simulink model "Torque_Control_ETR07"  (R2017b)
settings: Solver=FixedStepAuto  StartTime=0.0  StopTime=10.0  RelTol=1e-3
libraries: simulink x15, dspstat3 x1
(part 2 of 5)

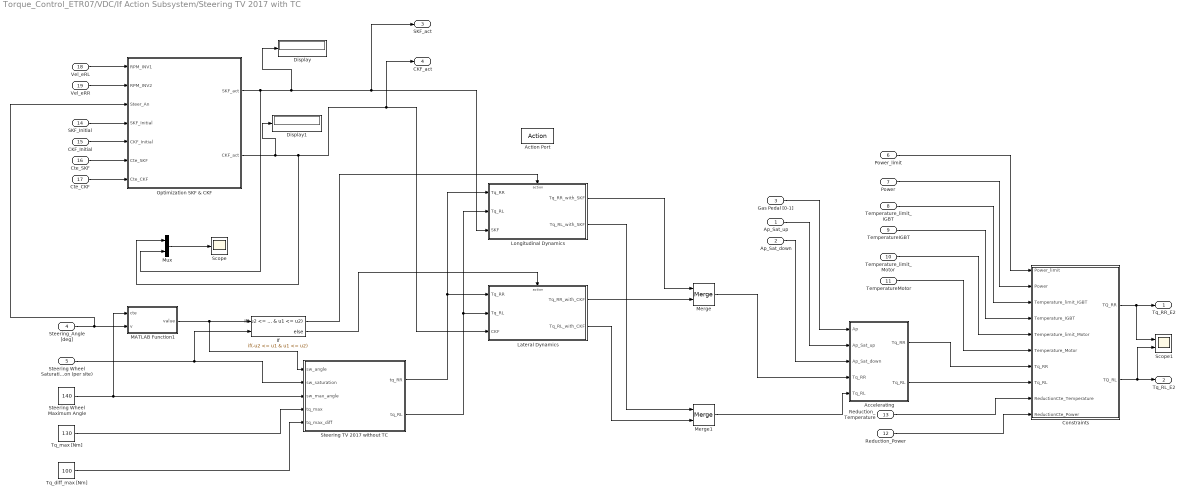
== system Torque_Control_ETR07/VDC/If Action Subsystem/Steering TV 2017 with TC ==
  "Ap_Sat_up " : Inport
  Ap_Sat_down : Inport  Port=2
  Gas Pedal [0-1] : Inport  Port=3
  Steering_Angle [deg] : Inport  Port=4
  "Steering Wheel Saturation (per site) " : Inport  Port=5
  Power_limit : Inport  Port=6
  Power : Inport  Port=7
  Temperature_limit_IGBT : Inport  Port=8
  TemperatureIGBT : Inport  Port=9
  Temperature_limit_Motor : Inport  Port=10
  TemperatureMotor : Inport  Port=11
  Reduction_Power : Inport  Port=12
  Reduction_Temperature : Inport  Port=13
  SKF_Initial : Inport  Port=14
  CKF_Initial : Inport  Port=15
  Cte_SKF : Inport  Port=16
  Cte_CKF : Inport  Port=17
  Vel_eRL : Inport  Port=18
  Vel_eRR : Inport  Port=19
  Action Port : ActionPort  ActionType=elseif
  Accelerating : Subsystem
  Constraints : Subsystem
  Display : Display
  Display1 : Display
  If : If  NumInputs=2  IfExpression=-u2 <= u1 & u1 <= u2
  Lateral Dynamics : Subsystem  TreatAsAtomicUnit=on
  Longitudinal Dynamics : Subsystem  TreatAsAtomicUnit=on
  MATLAB Function1 : MATLAB Function  TreatAsAtomicUnit=on
  Merge : Merge
  Merge1 : Merge
  Mux : Mux  Inputs=2
  Optimization SKF & CKF : Subsystem
  Scope : Scope
  Scope1 : Scope  NumInputPorts=2
  Steering TV 2017 without TC : MATLAB Function  TreatAsAtomicUnit=on
  Steering Wheel Maximum Angle : Constant  Value=140
  Tq_diff_max [Nm] : Constant  Value=100
  Tq_max [Nm] : Constant  Value=130
  Tq_RR_E2 : Outport
  Tq_RL_E2 : Outport  Port=2
  SKF_act : Outport  Port=3
  CKF_act : Outport  Port=4
  wires:
  Gas Pedal [0-1]/1 -> Accelerating/1(Ap)
  "Ap_Sat_up "/1 -> Accelerating/2("Ap_Sat_up ")
  Ap_Sat_down/1 -> Accelerating/3(Ap_Sat_down)
  Tq_max [Nm]/1 -> Steering TV 2017 without TC/4(tq_max)
  Tq_diff_max [Nm]/1 -> Steering TV 2017 without TC/5(tq_max_diff)
  Steering Wheel Maximum Angle/1 -> Steering TV 2017 without TC/3(sw_max_angle), MATLAB Function1/1(cte)
  "Steering Wheel Saturation (per site) "/1 -> If/2, Steering TV 2017 without TC/2(sw_saturation)
  Steering TV 2017 without TC/1(tq_RR) -> Lateral Dynamics/1(Tq_RR), Longitudinal Dynamics/1(Tq_RR)
  Steering TV 2017 without TC/2(tq_RL) -> Lateral Dynamics/2(Tq_RL), Longitudinal Dynamics/2(Tq_RL)
  Power_limit/1 -> Constraints/1(Power_limit)
  Power/1 -> Constraints/2(Power)
  Temperature_limit_IGBT/1 -> Constraints/3(Temperature_limit_IGBT)
  TemperatureIGBT/1 -> Constraints/4(Temperature_IGBT)
  Reduction_Temperature/1 -> Constraints/9(ReductionCte_Temperature)
  Reduction_Power/1 -> Constraints/10(ReductionCte_Power)
  Constraints/1(TQ_RR) -> Scope1/1, Tq_RR_E2/1
  Constraints/2(TQ_RL) -> Scope1/2, Tq_RL_E2/1
  Accelerating/2(Tq_RL) -> Constraints/8(Tq_RL)
  Accelerating/1("Tq_RR ") -> Constraints/7(Tq_RR)
  MATLAB Function1/1(value) -> Steering TV 2017 without TC/1(sw_angle), If/1
  Temperature_limit_Motor/1 -> Constraints/5(Temperature_limit_Motor)
  TemperatureMotor/1 -> Constraints/6(Temperature_Motor)
  Optimization SKF & CKF/2(CKF_act) -> Display1/1, Mux/1, Lateral Dynamics/3(CKF), CKF_act/1
  SKF_Initial/1 -> Optimization SKF & CKF/4(SKF_Initial)
  Mux/1 -> Scope/1
  Cte_SKF/1 -> Optimization SKF & CKF/6(Cte_SKF)
  Vel_eRL/1 -> Optimization SKF & CKF/1(RPM_INV1)
  Vel_eRR/1 -> Optimization SKF & CKF/2(RPM_INV2)
  Optimization SKF & CKF/1(SKF_act) -> SKF_act/1, Longitudinal Dynamics/3(SKF), Display/1, Mux/2
  Steering_Angle [deg]/1 -> MATLAB Function1/2(v), Optimization SKF & CKF/3(Steer_An)
  CKF_Initial/1 -> Optimization SKF & CKF/5(CKF_Initial)
  Cte_CKF/1 -> Optimization SKF & CKF/7(Cte_CKF)
  If/1 -> Longitudinal Dynamics/Action
  Lateral Dynamics/2(Tq_RL_with_CKF) -> Merge1/2
  If/2 -> Lateral Dynamics/Action
  Longitudinal Dynamics/2(Tq_RL_with_SKF) -> Merge1/1
  Longitudinal Dynamics/1(Tq_RR_with_SKF) -> Merge/1
  Lateral Dynamics/1(Tq_RR_with_CKF) -> Merge/2
  Merge/1 -> Accelerating/4(Tq_RR)
  Merge1/1 -> Accelerating/5("Tq_RL ")

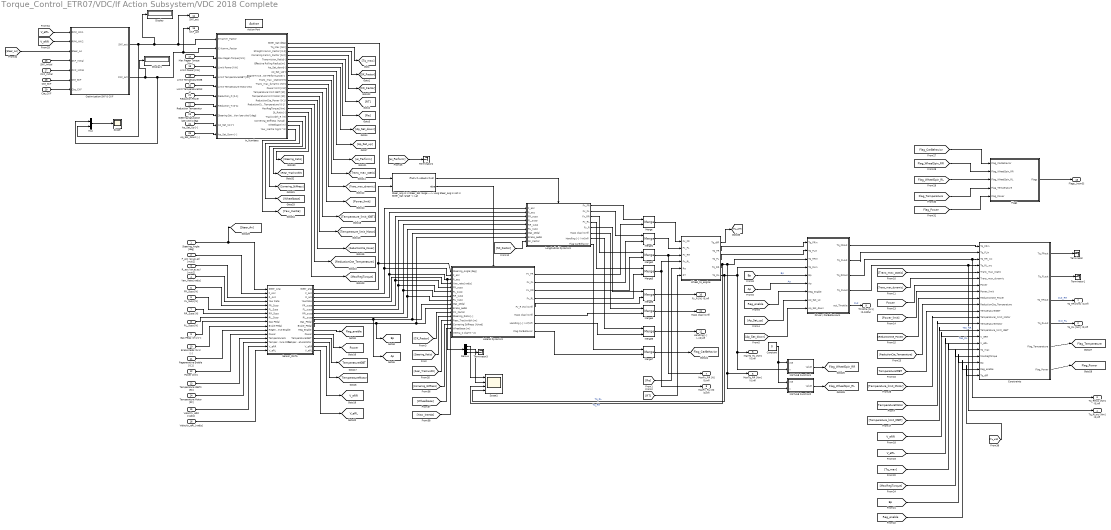
== system Torque_Control_ETR07/VDC/If Action Subsystem/VDC 2018 Complete ==
  Steering_Angle [deg] : Inport
  F_acc (ax,ay,az) [m/s2] : Inport  Port=2
  R_acc (ax,ay,az) [m/s2] : Inport  Port=3
  Yaw_Rate [rad/s] : Inport  Port=4
  FR_Susp [N] : Inport  Port=5
  FL_Susp [N] : Inport  Port=6
  RR_Susp [N] : Inport  Port=7
  RL_Susp [N] : Inport  Port=8
  Gas Pedal (0-1) [-] : Inport  Port=9
  Brake Pedal (0-1) [-] : Inport  Port=10
  Regenerative Enable [0,1] : Inport  Port=11
  Power [kW] : Inport  Port=12
  Temperature IGBTs [ºC] : Inport  Port=13
  Temperature Motor [ºC] : Inport  Port=14
  Velocity_eRR [rad/s] : Inport  Port=15
  Velocity_eRL [rad/s] : Inport  Port=16
  Max Regen Torque [Nm] : Inport  Port=17
  Limit Power [kW] : Inport  Port=18
  Limit TemperatureIGBT : Inport  Port=19
  Limit TemperatureMotor : Inport  Port=20
  Reduction Power : Inport  Port=21
  Reduction Temperature : Inport  Port=22
  Steering Saturation (per site) [deg] : Inport  Port=23
  Ap_Sat_Up [-] : Inport  Port=24
  Ap_Sat_Down [-] : Inport  Port=25
  SKF_Initial : Inport  Port=26
  CKF_Initial : Inport  Port=27
  Cte_SKF : Inport  Port=28
  Cte_CKF : Inport  Port=29
  Action Port : ActionPort  ActionType=then
  Constant : Constant  Value=0
  Constraints : Subsystem
  Demux : Demux  Outputs=3
  Display : Display
  Display1 : Display
  Driver / CarBehaviours : Subsystem
  Flags : Subsystem
  In_Numbers : Subsystem
  Lateral Dynamics : Subsystem  TreatAsAtomicUnit=on
  Longitudinal Dynamics : Subsystem  TreatAsAtomicUnit=on
  MATLAB Function1 : MATLAB Function  TreatAsAtomicUnit=on
  MATLAB Function2 : MATLAB Function  TreatAsAtomicUnit=on
  Merge{,1..7} (8 alike) : Merge
  Mux : Mux  Inputs=2
  Optimization SKF & CKF : Subsystem
  Scope : Scope
  Scope1 : Scope  NumInputPorts=4
  Sensor_DATA : Subsystem
  "Steer_ang is in Steer_Sat range ---> Long Steer_ang is not in Steer_Sat range -> Lat " : If  NumInputs=2  IfExpression=u2>=-u1&u2<=u1
  Terminator{,1..3} (4 alike) : Terminator
  Wheel_to_engine : Subsystem
  Tq_RR [Nm] (0,inf) : Outport
  Tq_RL [Nm] (0,inf) : Outport  Port=2
  Tq_RRwc [Nm] (0,inf) : Outport  Port=3
  Tq_RLwc [Nm] (0,inf) : Outport  Port=4
  MaxTq_RR [Nm] (0,inf) : Outport  Port=5
  MaxTq_RL [Nm] (0,inf) : Outport  Port=6
  MaxFx_RR [N] (0,inf) : Outport  Port=7
  MaxFx_RL [N] (0,inf) : Outport  Port=8
  Throttle [0-1] (0-100%) : Outport  Port=9
  Fy_R [N] (0,inf) : Outport  Port=10
  Mass [kg] (0,inf) : Outport  Port=11
  Handling [-] (-inf,inf) : Outport  Port=12
  Flags_[num5] : Outport  Port=13
  SKF_act : Outport  Port=14
  CKF_act : Outport  Port=15
  tag scope: Ap=global, Bp=global, Flag_CarBehavior=global, Flag_Power=global, Flag_Temperature=global, Flag_WheelSpin_RL=global, Flag_WheelSpin_RR=global, Power=global, Reg_enable=global, TemperatureIGBT=global, TemperatureMotor=global, V_eRL=global, V_eRR=global
  wires:
  "Steer_ang is in Steer_Sat range ---> Long Steer_ang is not in Steer_Sat range -> Lat "/1 -> Longitudinal Dynamics/Action
  "Steer_ang is in Steer_Sat range ---> Long Steer_ang is not in Steer_Sat range -> Lat "/2 -> Lateral Dynamics/Action
  Sensor_DATA/8(RL_susp) -> Longitudinal Dynamics/6(RL_susp), Lateral Dynamics/8(RL_susp)
  In_Numbers/3(Straight Kamm_Factor [0-2]) -> [SK_Factor]
  In_Numbers/1(Steer_Sat [deg]) -> "Steer_ang is in Steer_Sat range ---> Long Steer_ang is not in Steer_Sat range -> Lat "/1
  In_Numbers/2(Tq_Max [Nm]) -> [Tq_max]
  Sensor_DATA/9(Gas_Pedal) -> [Ap], Lateral Dynamics/9(Gas_pedal), Longitudinal Dynamics/7(Gas_pedal)
  In_Numbers/6(Effective Rolling Radius[m]) -> [Re]
  In_Numbers/5(Transmision_Ratio[-]) -> [RT]
  Sensor_DATA/7(RR_susp) -> Longitudinal Dynamics/5(RR_susp), Lateral Dynamics/7(RR_susp)
  In_Numbers/8(Ap_Sat_up[-]) -> [Ap_Sat_up]
  In_Numbers/7(Ap_Sat_down[-]) -> [Ap_Sat_down]
  Driver / CarBehaviours/3(Tq_RRout) -> Tq_RRwc [Nm] (0,inf)/1, Constraints/3(Tq_RR_wc)  "Teo_RR"
  Sensor_DATA/2(F_acc) -> Longitudinal Dynamics/1(F_acc), Lateral Dynamics/2(F_acc)
  Sensor_DATA/3(R_acc) -> Longitudinal Dynamics/2(R_acc), Demux/1, Lateral Dynamics/3(R_acc)
  Sensor_DATA/10(Brake_Pedal) -> [Bp], Lateral Dynamics/10(Brake_pedal), Longitudinal Dynamics/8(Brake_pedal)
  Sensor_DATA/6(FL_susp) -> Longitudinal Dynamics/4(FL_susp), Lateral Dynamics/6(FL_susp)
  Sensor_DATA/11(Reg_Enable) -> [Reg_enable]
  Sensor_DATA/5(FR_susp) -> Longitudinal Dynamics/3(FR_susp), Lateral Dynamics/5(FR_susp)
  Sensor_DATA/1(Steer_ang) -> Lateral Dynamics/1(Steering_Angle [deg]), "Steer_ang is in Steer_Sat range ---> Long Steer_ang is not in Steer_Sat range -> Lat "/2
  Wheel_to_engine/5(Tq_RL) -> Scope1/4, MaxTq_RL [Nm] (0,inf)/1, MATLAB Function1/2(v), Driver / CarBehaviours/4("Tq_RLin ")  "Tq_RL"
  [Trans_max_dynamic] -> Constraints/6(Trans_max_dynamic)
  [Power_limit] -> Constraints/8(Power_limit)
  In_Numbers/15(ReductionCte_Power (0-1)) -> [ReductionCte_Power]
  Driver / CarBehaviours/5(out_Throttle) -> Throttle [0-1] (0-100%)/1  "Out"
  Wheel_to_engine/4(Tq_RR) -> Scope1/3, MATLAB Function2/2(v), MaxTq_RR [Nm] (0,inf)/1, Driver / CarBehaviours/3(Tq_RRin)  "Tq_RR"
  Wheel_to_engine/3(Tq_FL) -> Driver / CarBehaviours/2(Tq_FLin)
  In_Numbers/11(Trans_max_dynamic [Nm]) -> [Trans_max_dynamic]
  [Reg_enable] -> Driver / CarBehaviours/7(Reg_enable)
  [ReductionCte_Power] -> Constraints/9(ReductionCte_Power)
  [Ap_Sat_up] -> Driver / CarBehaviours/8(Ap_Sat_up)
  In_Numbers/10(Trans_max _static[Nm]) -> [Trans_max_static]
  [Ap] -> Driver / CarBehaviours/6(Ap)  "Ap"
  [Power] -> Constraints/7(Power)
  In_Numbers/12("Power limit [KW] ") -> [Power_limit]
  [Ap_Sat_down] -> Driver / CarBehaviours/9(Ap_Sat_down)
  Driver / CarBehaviours/4(Tq_RLout) -> Tq_RLwc [Nm] (0,inf)/1, Constraints/4("Tq_RL_wc ")  "Teo_RL"
  Driver / CarBehaviours/2("Tq_FLout ") -> Constraints/2(Tq_FLin)
  Steering_Angle [deg]/1 -> [Steer_An], Sensor_DATA/1(Steer_Ang)
  Wheel_to_engine/2(Tq_FR) -> Driver / CarBehaviours/1(Tq_FRin)
  Driver / CarBehaviours/1(Tq_FRout) -> Constraints/1(Tq_FRin)
  [Trans_max_static] -> Constraints/5("Trans_max_static ")
  [Temperature_limit_IGBT] -> Constraints/14(Temperature_limit_IGBT)
  [Bp] -> Constraints/19(Bp)
  Sensor_DATA/16(V_eRL) -> [V_eRL]
  In_Numbers/17(MaxRegTorque [Nm]) -> [MaxRegTorque]
  [TemperatureIGBT] -> Constraints/11(TemperatureIGBT)
  [Reg_enable] -> Constraints/20(Reg_enable)
  In_Numbers/9(Engine+Inverter Performance[-]) -> [ei_Perform]
  [Bp] -> Driver / CarBehaviours/5(Bp)  "Bp"
  [Tq_max] -> Constraints/17(Tq_max)
  RR_Susp [N]/1 -> Sensor_DATA/7(RR_Susp)
  Power [kW]/1 -> Sensor_DATA/12("Power ")
  Sensor_DATA/12(Power) -> [Power]
  Sensor_DATA/15("V_eRR ") -> [V_eRR]
  [V_eRR] -> Constraints/15(V_eRR)
  Regenerative Enable [0,1]/1 -> Sensor_DATA/11(Regenerative Enable)
  Brake Pedal (0-1) [-]/1 -> Sensor_DATA/10(Brake Pedal)
  [V_eRL] -> Constraints/16(V_eRL)
  In_Numbers/13(Temperature limit IGBT [ºC]) -> [Temperature_limit_IGBT]
  FL_Susp [N]/1 -> Sensor_DATA/6(FL_Susp)
  FR_Susp [N]/1 -> Sensor_DATA/5(FR_Susp)
  R_acc (ax,ay,az) [m/s2]/1 -> Sensor_DATA/3(R_Acc)
  F_acc (ax,ay,az) [m/s2]/1 -> Sensor_DATA/2("F_Acc ")
  RL_Susp [N]/1 -> Sensor_DATA/8(RL_Susp)
  Gas Pedal (0-1) [-]/1 -> Sensor_DATA/9(Gas Pedal)
  Temperature IGBTs [ºC]/1 -> Sensor_DATA/13(TemperatureIN)
  Velocity_eRR [rad/s]/1 -> Sensor_DATA/15(V_eRR)
  Velocity_eRL [rad/s]/1 -> Sensor_DATA/16("V_eRL ")
  Constraints/1(Tq_FRout) -> Terminator/1
  Constraints/2("Tq_FLout ") -> Terminator1/1
  In_Numbers/4(Cornering Kamm_Factor [0-2]) -> [CK_Factor]
  [Re] -> Wheel_to_engine/5(Re)
  [RT] -> Wheel_to_engine/6(RT)
  Merge3/1 -> MaxFx_RL [N] (0,inf)/1, Wheel_to_engine/4("Fx_RL ")
  Merge2/1 -> Wheel_to_engine/3("Fx_RR "), MaxFx_RR [N] (0,inf)/1
  Merge1/1 -> Wheel_to_engine/2("Fx_FL ")
  Max Regen Torque [Nm]/1 -> In_Numbers/3(Max Regen Torque [Nm])
  Limit Power [kW]/1 -> In_Numbers/4(Limit Power [kW])
  Limit TemperatureIGBT/1 -> In_Numbers/5(Limit TemperatureIGBT [ºC])
  Reduction Power/1 -> In_Numbers/7(Reduction_P [0-1])
  [CK_Factor] -> Lateral Dynamics/11(CK_Factor)
  [SK_Factor] -> Longitudinal Dynamics/9(SK_Factor)
  Longitudinal Dynamics/1(Fx_FR) -> Merge/1
  Longitudinal Dynamics/2(Fx_FL) -> Merge1/1
  Longitudinal Dynamics/3("Fx_RR ") -> Merge2/1
  Longitudinal Dynamics/4("Fx_RL ") -> Merge3/1
  Lateral Dynamics/1(Fx_FR) -> Merge/2
  Lateral Dynamics/2(Fx_FL) -> Merge1/2
  Lateral Dynamics/3("Fx_RR ") -> Merge2/2
  Lateral Dynamics/4("Fx_RL ") -> Merge3/2
  Merge/1 -> Wheel_to_engine/1("Fx_FR ")
  Steering Saturation (per site) [deg]/1 -> In_Numbers/9(Steering Saturation (per site) [deg])
  Ap_Sat_Up [-]/1 -> In_Numbers/10(Ap_Sat_Up [-])
  Ap_Sat_Down [-]/1 -> In_Numbers/11(Ap_Sat_Down [-])
  [MaxRegTorque] -> Constraints/18(MaxRegTorque)
  [ei_Perform] -> Terminator2/1
  Merge4/1 -> Mass [kg] (0,inf)/1
  Longitudinal Dynamics/6(Mass [kg] (0,inf)) -> Merge4/1
  Lateral Dynamics/6(" Mass [kg] (0,inf)") -> Merge4/2
  Longitudinal Dynamics/7(Handling [-] (-inf,inf)) -> Merge5/1
  Lateral Dynamics/7(Handling [-] (-inf,inf)) -> Merge5/2
  Merge5/1 -> Handling [-] (-inf,inf)/1
  Merge6/1 -> Fy_R [N] (0,inf)/1
  Lateral Dynamics/5(Fy_R [N] (0,inf)) -> Merge6/2
  Longitudinal Dynamics/5(Fy_R) -> Merge6/1
  In_Numbers/16(ReductionCte_Temperature (0-1)) -> [ReductionCte_Temperature]
  Reduction Temperature/1 -> In_Numbers/8(Reduction_T [0-1])
  [ReductionCte_Temperature] -> Constraints/10(ReductionCte_Temperature)
  Constraints/3(Tq_RRout) -> Tq_RR [Nm] (0,inf)/1  "Out_RR"
  Constraints/4(Tq_RLout) -> Tq_RL [Nm] (0,inf)/1  "Out_RL"
  Temperature Motor [ºC]/1 -> Sensor_DATA/14(Temperature Motor)
  Sensor_DATA/13(TemperatureIGBT) -> [TemperatureIGBT]
  Sensor_DATA/14(TemperatureMotor) -> [TemperatureMotor]
  [TemperatureMotor] -> Constraints/13(TemperatureIMotor)
  [Temperature_limit_Motor] -> Constraints/12(TemperatureI_limit_Motor)
  In_Numbers/14(Temperature limit Motor [ºC]) -> [Temperature_limit_Motor]
  Limit TemperatureMotor/1 -> In_Numbers/6(Limit Temperature Motor [ºC])
  Merge7/1 -> [Flag_CarBehavior]
  Longitudinal Dynamics/8(Flag CarBehavior) -> Merge7/1
  Lateral Dynamics/8(Flag CarBehavior) -> Merge7/2
  MATLAB Function2/1(value) -> [Flag_WheelSpin_RL]
  MATLAB Function1/1(value) -> [Flag_WheelSpin_RR]
  Constant/1 -> MATLAB Function2/1(cte), MATLAB Function1/1(cte)
  Constraints/5(Flag_Temperature) -> [Flag_Temperature]
  Constraints/6(Flag_Power) -> [Flag_Power]
  Flags/1(Flags) -> Flags_[num5]/1
  [Flag_WheelSpin_RL] -> Flags/3(Flag_WheelSpin_RL)
  [Flag_WheelSpin_RR] -> Flags/2(Flag_WheelSpin_RR)
  [Flag_CarBehavior] -> Flags/1(Flag_CarBehavior)
  [Flag_Temperature] -> Flags/4(Flag_Temperature)
  [Flag_Power] -> Flags/5(Flag_Power)
  Optimization SKF & CKF/1(SKF_act) -> In_Numbers/1(S-Kamm_Factor), SKF_act/1, Display/1, Mux/2
  CKF_Initial/1 -> Optimization SKF & CKF/5(CKF_Initial)
  [Steer_An] -> Optimization SKF & CKF/3(Steer_An)
  [V_eRR] -> Optimization SKF & CKF/2(RPM_INV2)
  Cte_SKF/1 -> Optimization SKF & CKF/6(Cte_SKF)
  Cte_CKF/1 -> Optimization SKF & CKF/7(Cte_CKF)
  SKF_Initial/1 -> Optimization SKF & CKF/4(SKF_Initial)
  [V_eRL] -> Optimization SKF & CKF/1(RPM_INV1)
  Optimization SKF & CKF/2(CKF_act) -> Display1/1, Mux/1, In_Numbers/2(C-Kamm_Factor), CKF_act/1
  Mux/1 -> Scope/1
  Yaw_Rate [rad/s]/1 -> Sensor_DATA/4(Yaw Rate)
  Sensor_DATA/4(YawRate) -> Lateral Dynamics/4(Yaw_rate [rad/s])
  In_Numbers/18(St_Ratio [-]) -> [Steering_Ratio]
  [Steering_Ratio] -> Lateral Dynamics/12(Steering_Ratio [-])
  Demux/2 -> Scope1/2
  Demux/1 -> Scope1/1
  Demux/3 -> Terminator3/1
  In_Numbers/19(Trackwidth_R (m)) -> [Rear_Trackwidth]
  In_Numbers/20(Cornering_Stiffness (N/rad)) -> [Cornering_Stiffness]
  In_Numbers/21(Wheelbase (m)) -> [Wheelbase]
  [Rear_Trackwidth] -> Lateral Dynamics/13(Rear_Trackwidth [m])
  [Cornering_Stiffness] -> Lateral Dynamics/14(Cornering Stiffness [N/rad])
  [Wheelbase] -> Lateral Dynamics/15(Wheelbase [m])
  In_Numbers/22(Yaw_Inertia (kg/m^3)) -> [Yaw_Inertia]
  [Yaw_Inertia] -> Lateral Dynamics/16(Inertia_Z [kg*m^2])
  Wheel_to_engine/1(Tq_diff) -> [Tq_diff]
  [Tq_diff] -> Constraints/21(Tq_diff)

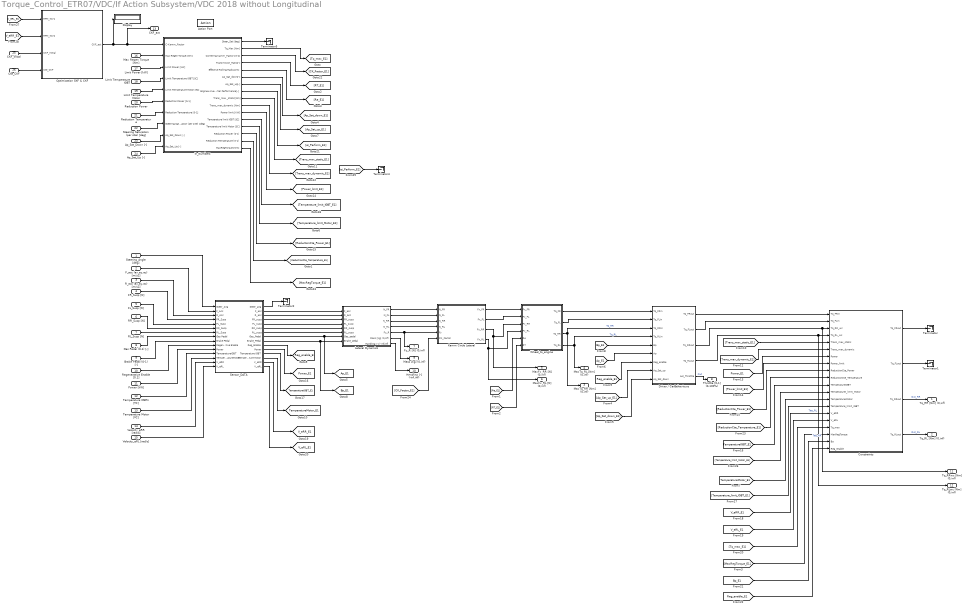
== system Torque_Control_ETR07/VDC/If Action Subsystem/VDC 2018 without Longitudinal ==
  Steering_Angle [deg] : Inport
  F_acc (ax,ay,az) [m/s2] : Inport  Port=2
  R_acc (ax,ay,az) [m/s2] : Inport  Port=3
  FR_Susp [N] : Inport  Port=4
  FL_Susp [N] : Inport  Port=5
  RR_Susp [N] : Inport  Port=6
  RL_Susp [N] : Inport  Port=7
  Gas Pedal (0-1) [-] : Inport  Port=8
  Brake Pedal (0-1) [-] : Inport  Port=9
  Regenerative Enable [0,1] : Inport  Port=10
  Power [kW] : Inport  Port=11
  Temperature IGBTs [ºC] : Inport  Port=12
  Temperature Motor [ºC] : Inport  Port=13
  Velocity_eRR [rad/s] : Inport  Port=14
  Velocity_eRL [rad/s] : Inport  Port=15
  Max Regen Torque [Nm] : Inport  Port=16
  Limit Power [kW] : Inport  Port=17
  Limit Temperature IGBT : Inport  Port=18
  Limit Temperature Motor : Inport  Port=19
  Reduction Power : Inport  Port=20
  Reduction Temperature : Inport  Port=21
  Steering Saturation (per site) [deg] : Inport  Port=22
  Ap_Sat_Down [-] : Inport  Port=23
  Ap_Sat_Up [-] : Inport  Port=24
  CKF_Initial : Inport  Port=25
  Cte_CKF : Inport  Port=26
  Action Port : ActionPort  ActionType=elseif
  Constraints : Subsystem
  Display : Display
  Driver / CarBehaviours : Subsystem
  In_Numbers : Subsystem
  Kamm Circle Lateral : Subsystem
  Lateral Dynamics : Subsystem
  Optimization SKF & CKF : Subsystem
  Sensor_DATA : Subsystem
  Terminator{,1..2,4..5} (5 alike) : Terminator
  Wheel_to_engine : Subsystem
  Tq_RR [Nm] (0,inf) : Outport
  Tq_RL [Nm] (0,inf) : Outport  Port=2
  MaxTq_RR [Nm] (0,inf) : Outport  Port=3
  MaxTq_RL [Nm] (0,inf) : Outport  Port=4
  MaxFx_RR [N] (0,inf) : Outport  Port=5
  MaxFx_RL [N] (0,inf) : Outport  Port=6
  Fy_R [N] (0,inf) : Outport  Port=7
  Throttle [0-1] (0-100%) : Outport  Port=8
  Mass [kg] (0,inf) : Outport  Port=9
  Handling [-] (-inf,inf) : Outport  Port=10
  Tq_RRwc [Nm] (0,inf) : Outport  Port=11
  Tq_RLwc [Nm] (0,inf) : Outport  Port=12
  CKF_act : Outport  Port=13
  tag scope: Ap_E1=global, Bp_E1=global, Power_E1=global, Reg_enable_E1=global, TemperatureIGBT_E1=global, TemperatureMotor_E1=global, V_eRL_E1=global, V_eRR_E1=global
  wires:
  Sensor_DATA/7(RL_susp) -> Lateral Dynamics/6(RL_susp)
  In_Numbers/2(Tq_Max [Nm]) -> [Tq_max_E1]
  Sensor_DATA/8(Gas_Pedal) -> [Ap_E1], Lateral Dynamics/7(Gas_pedal)
  In_Numbers/5(Effective Rolling Radius[m]) -> [Re_E1]
  In_Numbers/4(Transmision_Ratio[-]) -> [RT_E1]
  Sensor_DATA/6(RR_susp) -> Lateral Dynamics/5(RR_susp)
  In_Numbers/7(Ap_Sat_up[-]) -> [Ap_Sat_up_E1]
  In_Numbers/6(Ap_Sat_down[-]) -> [Ap_Sat_down_E1]
  Sensor_DATA/2(F_acc) -> Lateral Dynamics/1(F_acc)
  Sensor_DATA/3(R_acc) -> Lateral Dynamics/2(R_acc)
  Sensor_DATA/9(Brake_Pedal) -> [Bp_E1], Lateral Dynamics/8(Brake_pedal)
  Sensor_DATA/5(FL_susp) -> Lateral Dynamics/4(FL_susp)
  Sensor_DATA/10(Reg_Enable) -> [Reg_enable_E1]
  Sensor_DATA/4(FR_susp) -> Lateral Dynamics/3(FR_susp)
  Wheel_to_engine/4(Tq_RL) -> MaxTq_RL [Nm] (0,inf)/1, Driver / CarBehaviours/4("Tq_RLin ")  "Tq_RL"
  In_Numbers/14(Reduction Power (0-1)) -> [ReductionCte_Power_E1]
  Wheel_to_engine/3(Tq_RR) -> MaxTq_RR [Nm] (0,inf)/1, Driver / CarBehaviours/3(Tq_RRin)  "Tq_RR"
  Wheel_to_engine/2(Tq_FL) -> Driver / CarBehaviours/2(Tq_FLin)
  In_Numbers/10(Trans_max_dynamic [Nm]) -> [Trans_max_dynamic_E1]
  [Reg_enable_E1] -> Driver / CarBehaviours/7(Reg_enable)
  [Ap_Sat_up_E1] -> Driver / CarBehaviours/8(Ap_Sat_up)
  In_Numbers/9(Trans_max _static[Nm]) -> [Trans_max_static_E1]
  [Ap_E1] -> Driver / CarBehaviours/6(Ap)
  In_Numbers/11("Power limit [KW] ") -> [Power_limit_E1]
  [Ap_Sat_down_E1] -> Driver / CarBehaviours/9(Ap_Sat_down)
  Steering_Angle [deg]/1 -> Sensor_DATA/1(Steer_Ang)
  Wheel_to_engine/1(Tq_FR) -> Driver / CarBehaviours/1(Tq_FRin)
  Sensor_DATA/15(V_eRL) -> [V_eRL_E1]
  In_Numbers/16(MaxRegTorque [Nm]) -> [MaxRegTorque_E1]
  In_Numbers/8(Engine+Inverter Performance[-]) -> [ei_Perform_E1]
  [Bp_E1] -> Driver / CarBehaviours/5(Bp)
  Sensor_DATA/12(Temperature IGBT) -> [TemperatureIGBT_E1]
  RR_Susp [N]/1 -> Sensor_DATA/6(RR_Susp)
  Power [kW]/1 -> Sensor_DATA/11("Power ")
  Sensor_DATA/11(Power) -> [Power_E1]
  Sensor_DATA/14("V_eRR ") -> [V_eRR_E1]
  Regenerative Enable [0,1]/1 -> Sensor_DATA/10(Regenerative Enable)
  Brake Pedal (0-1) [-]/1 -> Sensor_DATA/9(Brake Pedal)
  In_Numbers/12(Temperature limit IGBT [ºC]) -> [Temperature_limit_IGBT_E1]
  FL_Susp [N]/1 -> Sensor_DATA/5(FL_Susp)
  FR_Susp [N]/1 -> Sensor_DATA/4(FR_Susp)
  R_acc (ax,ay,az) [m/s2]/1 -> Sensor_DATA/3(R_Acc)
  F_acc (ax,ay,az) [m/s2]/1 -> Sensor_DATA/2("F_Acc ")
  RL_Susp [N]/1 -> Sensor_DATA/7(RL_Susp)
  Gas Pedal (0-1) [-]/1 -> Sensor_DATA/8(Gas Pedal)
  Temperature IGBTs [ºC]/1 -> Sensor_DATA/12(TemperatureIGBT)
  Velocity_eRR [rad/s]/1 -> Sensor_DATA/14(V_eRR)
  Velocity_eRL [rad/s]/1 -> Sensor_DATA/15("V_eRL ")
  Max Regen Torque [Nm]/1 -> In_Numbers/2(Max Regen Torque [Nm])
  Limit Power [kW]/1 -> In_Numbers/3(Limit Power [kW])
  Limit Temperature IGBT/1 -> In_Numbers/4(Limit Temperature IGBT [ºC])
  Reduction Power/1 -> In_Numbers/6(Reduction Power [0-1])
  In_Numbers/3(Cornering Kamm_Factor [0-2]) -> [CK_Factor_E1]
  [Re_E1] -> Wheel_to_engine/5(Re)
  [RT_E1] -> Wheel_to_engine/6(RT)
  Ap_Sat_Up [-]/1 -> In_Numbers/10(Ap_Sat_Up [-])
  Ap_Sat_Down [-]/1 -> In_Numbers/9(Ap_Sat_Down [-])
  Steering Saturation (per site) [deg]/1 -> In_Numbers/8(Steering Saturation (per site) [deg])
  [CK_Factor_E1] -> Kamm Circle Lateral/6(CK_Factor)
  Kamm Circle Lateral/1(Fx_FR) -> Wheel_to_engine/1("Fx_FR ")
  Kamm Circle Lateral/2(Fx_FL) -> Wheel_to_engine/2("Fx_FL ")
  Kamm Circle Lateral/3("Fx_RR ") -> MaxFx_RR [N] (0,inf)/1, Wheel_to_engine/3("Fx_RR ")
  Kamm Circle Lateral/4("Fx_RL ") -> MaxFx_RL [N] (0,inf)/1, Wheel_to_engine/4("Fx_RL ")
  Sensor_DATA/1(Steer_ang) -> Terminator2/1
  Lateral Dynamics/1(N_FR) -> Kamm Circle Lateral/1("N_FR ")
  Lateral Dynamics/2("N_FL ") -> Kamm Circle Lateral/2(N_FL)
  Lateral Dynamics/3("N_RR ") -> Kamm Circle Lateral/3(N_RR)
  Lateral Dynamics/4(N_RL) -> Kamm Circle Lateral/4(N_RL)
  Lateral Dynamics/5(Fy_R) -> Fy_R [N] (0,inf)/1, Kamm Circle Lateral/5(Fy)
  Driver / CarBehaviours/5(out_Throttle) -> Throttle [0-1] (0-100%)/1  "Out"
  [ei_Perform_E1] -> Terminator4/1
  In_Numbers/1(Steer_Sat [deg]) -> Terminator5/1
  Lateral Dynamics/6(Mass [kg] (0,inf)) -> Mass [kg] (0,inf)/1
  Lateral Dynamics/7(Handling [-] (-inf,inf)) -> Handling [-] (-inf,inf)/1
  In_Numbers/15(Reduction Temperature (0-1)) -> [ReductionCte_Temperature_E1]
  Reduction Temperature/1 -> In_Numbers/7(Reduction Temperature [0-1])
  Driver / CarBehaviours/3(Tq_RRout) -> Tq_RRwc [Nm] (0,inf)/1, Constraints/3(Tq_RR_wc)  "Teo_RR"
  [Trans_max_dynamic_E1] -> Constraints/6(Trans_max_dynamic)
  [Power_limit_E1] -> Constraints/8(Power_limit)
  [ReductionCte_Power_E1] -> Constraints/9(ReductionCte_Power)
  [Power_E1] -> Constraints/7(Power)
  Driver / CarBehaviours/4(Tq_RLout) -> Tq_RLwc [Nm] (0,inf)/1, Constraints/4("Tq_RL_wc ")  "Teo_RL"
  Driver / CarBehaviours/2("Tq_FLout ") -> Constraints/2(Tq_FLin)
  Driver / CarBehaviours/1(Tq_FRout) -> Constraints/1(Tq_FRin)
  [Trans_max_static_E1] -> Constraints/5("Trans_max_static ")
  [Temperature_limit_IGBT_E1] -> Constraints/14(Temperature_limit_IGBT)
  [Bp_E1] -> Constraints/19(Bp)
  [TemperatureIGBT_E1] -> Constraints/11(TemperatureIGBT)
  [Reg_enable_E1] -> Constraints/20(Reg_enable)
  [Tq_max_E1] -> Constraints/17(Tq_max)
  [V_eRR_E1] -> Constraints/15(V_eRR)
  [V_eRL_E1] -> Constraints/16(V_eRL)
  Constraints/1(Tq_FRout) -> Terminator/1
  Constraints/2("Tq_FLout ") -> Terminator1/1
  [MaxRegTorque_E1] -> Constraints/18(MaxRegTorque)
  [ReductionCte_Temperature_E1] -> Constraints/10(ReductionCte_Temperature)
  Constraints/3(Tq_RRout) -> Tq_RR [Nm] (0,inf)/1  "Out_RR"
  Constraints/4(Tq_RLout) -> Tq_RL [Nm] (0,inf)/1  "Out_RL"
  [TemperatureMotor_E1] -> Constraints/13(TemperatureIMotor)
  [Temperature_limit_Motor_E1] -> Constraints/12(TemperatureI_limit_Motor)
  Limit Temperature Motor/1 -> In_Numbers/5(Limit Temperature Motor [ºC])
  In_Numbers/13(Temperature limit Motor [ºC]) -> [Temperature_limit_Motor_E1]
  Temperature Motor [ºC]/1 -> Sensor_DATA/13(TemperatureMotor)
  Sensor_DATA/13(Temperature Motor) -> [TemperatureMotor_E1]
  [V_eRR_E1] -> Optimization SKF & CKF/2(RPM_INV2)
  CKF_Initial/1 -> Optimization SKF & CKF/3(CKF_Initial)
  Cte_CKF/1 -> Optimization SKF & CKF/4(Cte_CKF)
  Optimization SKF & CKF/1(CKF_act) -> Display/1, In_Numbers/1(C-Kamm_Factor), CKF_act/1
  [V_eRL_E1] -> Optimization SKF & CKF/1(RPM_INV1)

== system Torque_Control_ETR07/VDC/Regeneration_Enable/Braking ==
  Latched : Inport
  Action Port : ActionPort  ActionType=then
  Enable : Outport
  wires:
  Latched/1 -> Enable/1

== system Torque_Control_ETR07/VDC/Regeneration_Enable/BypassDecision  ==
  In1 : Inport
  Action Port : ActionPort  ActionType=then
  Out1 : Outport
  wires:
  In1/1 -> Out1/1

== system Torque_Control_ETR07/VDC/Regeneration_Enable/Not-Braking ==
  Cell_Temp_ºC : Inport
  Prev_State : Inport  Port=2
  Action Port : ActionPort  ActionType=else
  If : If  NumInputs=2  IfExpression=u1 > u2
  If1 : If  IfExpression=u1 == 1
  Low_Threshold : Subsystem  TreatAsAtomicUnit=on
  Merge : Merge
  Merge1 : Merge
  Not_Braking : Constant  Value=0
  Temp_LIMIT : Subsystem  TreatAsAtomicUnit=on
  Temp_OK : Subsystem  TreatAsAtomicUnit=on
  Upper_Threshold : Subsystem  TreatAsAtomicUnit=on
  Enable : Outport
  Temp_Enable : Outport  Port=2
  wires:
  Cell_Temp_ºC/1 -> If/1
  If/1 -> Temp_LIMIT/Action
  If/2 -> Temp_OK/Action
  Temp_LIMIT/1(Out1) -> Merge/1
  Temp_OK/1(Out1) -> Merge/2
  Merge/1 -> Temp_Enable/1
  Not_Braking/1 -> Enable/1
  Prev_State/1 -> If1/1
  If1/1 -> Upper_Threshold/Action
  If1/2 -> Low_Threshold/Action
  Upper_Threshold/1(Out1) -> Merge1/1
  Low_Threshold/1(Out1) -> Merge1/2
  Merge1/1 -> If/2

== system Torque_Control_ETR07/VDC/Regeneration_Enable/NotEnabled ==
  In1 : Inport
  Action Port : ActionPort  ActionType=else
  Out1 : Outport
  wires:
  In1/1 -> Out1/1

== system Torque_Control_ETR07/VDC/TEST_MODE_IN/BYPASS ==
  In1 : Inport
  In2 : Inport  Port=2
  In3 : Inport  Port=3
  In4 : Inport  Port=4
  Action Port : ActionPort  ActionType=else
  Out1 : Outport
  Out2 : Outport  Port=2
  Out3 : Outport  Port=3
  Out4 : Outport  Port=4
  wires:
  In1/1 -> Out1/1
  In2/1 -> Out2/1
  In3/1 -> Out3/1
  In4/1 -> Out4/1

== system Torque_Control_ETR07/VDC/TEST_MODE_IN/TEST_CONSTANTS ==
  Action Port : ActionPort  ActionType=then
  Constant{,1..3} (4 alike) : Constant  Value=800
  Out1 : Outport
  Out2 : Outport  Port=2
  Out3 : Outport  Port=3
  Out4 : Outport  Port=4
  wires:
  Constant/1 -> Out1/1
  Constant1/1 -> Out2/1
  Constant2/1 -> Out3/1
  Constant3/1 -> Out4/1

== system Torque_Control_ETR07/VDC/WORKSHOP_MODE_RESTRICTIONS/BYPASS ==
  In1 : Inport
  In2 : Inport  Port=2
  Action Port : ActionPort  ActionType=else
  Out1 : Outport
  Out2 : Outport  Port=2
  wires:
  In1/1 -> Out1/1
  In2/1 -> Out2/1

== system Torque_Control_ETR07/VDC/WORKSHOP_MODE_RESTRICTIONS/Torque_Reduction  ==
  In1 : Inport
  In2 : Inport  Port=2
  Action Port : ActionPort  ActionType=then
  Constant : Constant  Value=150
  Divide : Product  Inputs=*/
  Divide1 : Product  Inputs=*/
  Saturation : Saturate  UpperLimit=10  LowerLimit=-10
  Saturation1 : Saturate  UpperLimit=10  LowerLimit=-10
  Out1 : Outport
  Out2 : Outport  Port=2
  wires:
  Saturation/1 -> Out1/1
  Saturation1/1 -> Out2/1
  In1/1 -> Divide/1
  Divide/1 -> Saturation/1
  In2/1 -> Divide1/1
  Divide1/1 -> Saturation1/1
  Constant/1 -> Divide1/2, Divide/2

== system Torque_Control_ETR07/Accumulator Power/PowerLimitDetection/OK_OrLatch/Latched Error ==
  Action Port : ActionPort  ActionType=then
  Constant : Constant
  "Out " : Outport
  wires:
  Constant/1 -> "Out "/1

== system Torque_Control_ETR07/Accumulator Power/PowerLimitDetection/OK_OrLatch/OK ==
  Action Port : ActionPort  ActionType=else
  Constant : Constant  Value=0
  "Out " : Outport
  wires:
  Constant/1 -> "Out "/1

== system Torque_Control_ETR07/VDC/If Action Subsystem/Rigid Axle/Accelerating ==
  Ap : Inport
  "Ap_Sat_up " : Inport  Port=2
  Ap_Sat_down : Inport  Port=3
  Tq_RR : Inport  Port=4
  "Tq_RL " : Inport  Port=5
  "Accelerator behaviour " : MATLAB Function  TreatAsAtomicUnit=on
  Product : Product
  Product1 : Product
  "Tq_RR " : Outport
  Tq_RL : Outport  Port=2
  wires:
  Ap_Sat_down/1 -> "Accelerator behaviour "/3(Ap_Sat_down)
  Product/1 -> Tq_RL/1
  "Accelerator behaviour "/1(throttle) -> Product/1, Product1/1
  "Ap_Sat_up "/1 -> "Accelerator behaviour "/2(Ap_Sat_up)
  Ap/1 -> "Accelerator behaviour "/1(Ap)
  Tq_RR/1 -> Product1/2
  "Tq_RL "/1 -> Product/2
  Product1/1 -> "Tq_RR "/1

== system Torque_Control_ETR07/VDC/If Action Subsystem/Steering TV 2017 with TC/Accelerating ==
  Ap : Inport
  "Ap_Sat_up " : Inport  Port=2
  Ap_Sat_down : Inport  Port=3
  Tq_RR : Inport  Port=4
  "Tq_RL " : Inport  Port=5
  "Accelerator behaviour " : MATLAB Function  TreatAsAtomicUnit=on
  Product : Product
  Product1 : Product
  "Tq_RR " : Outport
  Tq_RL : Outport  Port=2
  wires:
  Ap_Sat_down/1 -> "Accelerator behaviour "/3(Ap_Sat_down)
  Product/1 -> Tq_RL/1
  "Accelerator behaviour "/1(throttle) -> Product/1, Product1/1
  "Ap_Sat_up "/1 -> "Accelerator behaviour "/2(Ap_Sat_up)
  Ap/1 -> "Accelerator behaviour "/1(Ap)
  Tq_RR/1 -> Product1/2
  "Tq_RL "/1 -> Product/2
  Product1/1 -> "Tq_RR "/1

== system Torque_Control_ETR07/VDC/If Action Subsystem/Steering TV 2017 with TC/Constraints ==
  note: Considero de la misma gravedad,
      | la limitacion por potencia que por temperatura
  Power_limit : Inport
  Power : Inport  Port=2
  Temperature_limit_IGBT : Inport  Port=3
  Temperature_IGBT : Inport  Port=4
  Temperature_limit_Motor : Inport  Port=5
  Temperature_Motor : Inport  Port=6
  Tq_RR : Inport  Port=7
  Tq_RL : Inport  Port=8
  ReductionCte_Temperature : Inport  Port=9
  ReductionCte_Power : Inport  Port=10
  "Control de Potencia " : Subsystem  TreatAsAtomicUnit=on
  Control de Temperatura : Subsystem  TreatAsAtomicUnit=on
  If : If  NumInputs=6  IfExpression=u4 >= u3 | u6 >= u5  ElseIfExpressions=u2 >= u1
  Merge : Merge  Inputs=3
  Merge1 : Merge  Inputs=3
  else : Subsystem  TreatAsAtomicUnit=on
  TQ_RR : Outport
  TQ_RL : Outport  Port=2
  wires:
  Temperature_IGBT/1 -> If/4
  ReductionCte_Power/1 -> "Control de Potencia "/3(ReductionCte)
  Power_limit/1 -> If/1
  Temperature_limit_IGBT/1 -> If/3
  ReductionCte_Temperature/1 -> Control de Temperatura/3(ReductionCte)
  Power/1 -> If/2
  "Control de Potencia "/1(Tq_RR_out) -> Merge/1
  "Control de Potencia "/2(Tq_RL_out) -> Merge1/1
  else/2(Tq_RL_out) -> Merge1/3
  If/1 -> Control de Temperatura/Action
  Tq_RR/1 -> else/1(Tq_RR), Control de Temperatura/1(Tq_RR), "Control de Potencia "/1(Tq_RR)
  Tq_RL/1 -> Control de Temperatura/2(Tq_RL), "Control de Potencia "/2(Tq_RL), else/2(Tq_RL)
  If/2 -> "Control de Potencia "/Action
  If/3 -> else/Action
  Control de Temperatura/1(Tq_RR_out) -> Merge/2
  else/1(Tq_RR_out) -> Merge/3
  Control de Temperatura/2(Tq_RL_out) -> Merge1/2
  Temperature_limit_Motor/1 -> If/5
  Temperature_Motor/1 -> If/6
  Merge/1 -> TQ_RR/1
  Merge1/1 -> TQ_RL/1

== system Torque_Control_ETR07/VDC/If Action Subsystem/Steering TV 2017 with TC/Lateral Dynamics ==
  Tq_RR : Inport
  Tq_RL : Inport  Port=2
  CKF : Inport  Port=3
  Action Port : ActionPort  ActionType=else
  Product : Product
  Product1 : Product
  Tq_RR_with_CKF : Outport
  Tq_RL_with_CKF : Outport  Port=2
  wires:
  Product1/1 -> Tq_RL_with_CKF/1
  Tq_RR/1 -> Product/1
  Tq_RL/1 -> Product1/1
  CKF/1 -> Product/2, Product1/2
  Product/1 -> Tq_RR_with_CKF/1

== system Torque_Control_ETR07/VDC/If Action Subsystem/Steering TV 2017 with TC/Longitudinal Dynamics ==
  Tq_RR : Inport
  Tq_RL : Inport  Port=2
  SKF : Inport  Port=3
  Action Port : ActionPort  ActionType=then
  Product : Product
  Product1 : Product
  Tq_RR_with_SKF : Outport
  Tq_RL_with_SKF : Outport  Port=2
  wires:
  Tq_RR/1 -> Product/1
  Tq_RL/1 -> Product1/1
  SKF/1 -> Product/2, Product1/2
  Product/1 -> Tq_RR_with_SKF/1
  Product1/1 -> Tq_RL_with_SKF/1

== system Torque_Control_ETR07/VDC/If Action Subsystem/Steering TV 2017 with TC/Optimization SKF & CKF ==
  RPM_INV1 : Inport
  RPM_INV2 : Inport  Port=2
  Steer_An : Inport  Port=3
  SKF_Initial : Inport  Port=4
  CKF_Initial : Inport  Port=5
  Cte_SKF : Inport  Port=6
  Cte_CKF : Inport  Port=7
  CKF_prev : DataStoreRead  DataStoreName=B
  Constant : Constant  Value=0
  Data Store Memory : DataStoreMemory  ReadBeforeWriteMsg=warning  WriteAfterWriteMsg=warning  WriteAfterReadMsg=warning  ShowAdditionalParam=off
  Data Store Memory1 : DataStoreMemory  DataStoreName=B  ReadBeforeWriteMsg=warning  WriteAfterWriteMsg=warning  WriteAfterReadMsg=warning  ShowAdditionalParam=off
  Data Store Write : DataStoreWrite
  Data Store Write1 : DataStoreWrite  DataStoreName=B
  Derivative : Derivative
  Display : Display
  MATLAB Function : MATLAB Function  TreatAsAtomicUnit=on
  Mux : Mux  Inputs=3
  "SKF_prev " : DataStoreRead
  Saturation : Saturate  UpperLimit=6000  LowerLimit=0
  Scope : Scope
  "Subsystem " : Subsystem
  Switch : Switch  Threshold=900
  SKF_act : Outport
  CKF_act : Outport  Port=2
  wires:
  SKF_Initial/1 -> "Subsystem "/3(SKF_Initial)
  CKF_prev/1 -> "Subsystem "/6("CKF_prev ")
  "Subsystem "/1("SKF_act ") -> SKF_act/1, Data Store Write/1  "SKF"
  Derivative/1 -> Switch/1, Switch/2, Saturation/1, Display/1, "Subsystem "/2(Derivative)  "alpha"
  "SKF_prev "/1 -> "Subsystem "/4(SKF_prev)
  "Subsystem "/2(CKF_act) -> CKF_act/1, Data Store Write1/1  "CKF"
  Cte_CKF/1 -> "Subsystem "/8(Cte_CKF)
  Steer_An/1 -> "Subsystem "/1(Steer_An)
  CKF_Initial/1 -> "Subsystem "/5("CKF_Initial ")
  RPM_INV1/1 -> Mux/1, MATLAB Function/1(RPM_INV1)
  RPM_INV2/1 -> MATLAB Function/2(RPM_INV2)
  Cte_SKF/1 -> "Subsystem "/7(Cte_SKF)
  MATLAB Function/1(RPM) -> Derivative/1  "w (rpm)"
  Mux/1 -> Scope/1
  Saturation/1 -> Mux/2
  Switch/1 -> Mux/3
  Constant/1 -> Switch/3

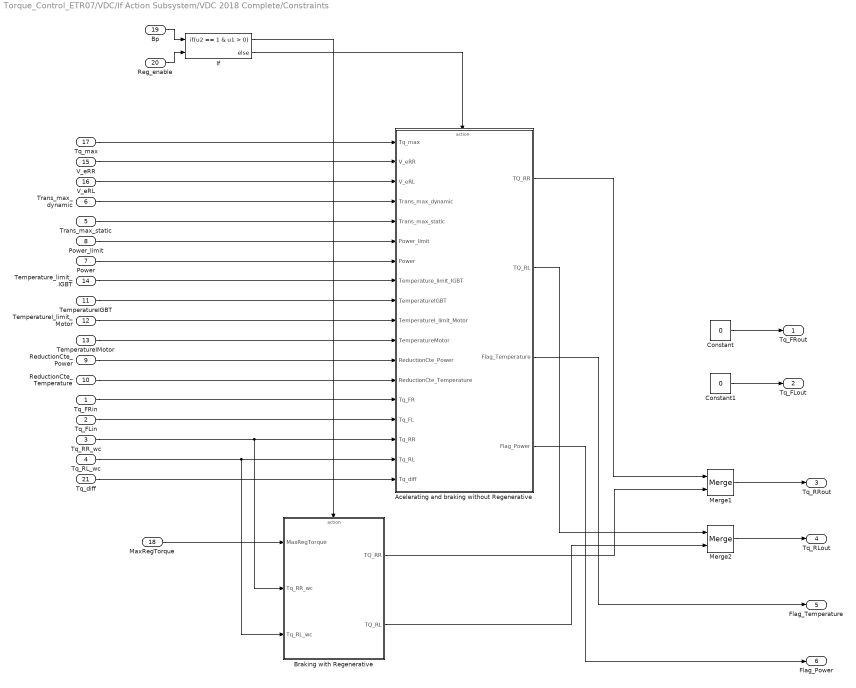
== system Torque_Control_ETR07/VDC/If Action Subsystem/VDC 2018 Complete/Constraints ==
  Tq_FRin : Inport
  Tq_FLin : Inport  Port=2
  Tq_RR_wc : Inport  Port=3
  "Tq_RL_wc " : Inport  Port=4
  "Trans_max_static " : Inport  Port=5
  Trans_max_dynamic : Inport  Port=6
  Power : Inport  Port=7
  Power_limit : Inport  Port=8
  ReductionCte_Power : Inport  Port=9
  ReductionCte_Temperature : Inport  Port=10
  TemperatureIGBT : Inport  Port=11
  TemperatureI_limit_Motor : Inport  Port=12
  TemperatureIMotor : Inport  Port=13
  Temperature_limit_IGBT : Inport  Port=14
  V_eRR : Inport  Port=15
  V_eRL : Inport  Port=16
  Tq_max : Inport  Port=17
  MaxRegTorque : Inport  Port=18
  Bp : Inport  Port=19
  Reg_enable : Inport  Port=20
  Tq_diff : Inport  Port=21
  Acelerating and braking without Regenerative : Subsystem  TreatAsAtomicUnit=on
  Braking with Regenerative : Subsystem  TreatAsAtomicUnit=on
  Constant : Constant  Value=0
  Constant1 : Constant  Value=0
  If : If  NumInputs=2  IfExpression=u2 == 1 & u1 > 0
  Merge1 : Merge
  Merge2 : Merge
  Tq_FRout : Outport
  "Tq_FLout " : Outport  Port=2
  Tq_RRout : Outport  Port=3
  Tq_RLout : Outport  Port=4
  Flag_Temperature : Outport  Port=5
  Flag_Power : Outport  Port=6
  wires:
  Constant1/1 -> "Tq_FLout "/1
  Constant/1 -> Tq_FRout/1
  Tq_RR_wc/1 -> Braking with Regenerative/2(Tq_RR_wc), Acelerating and braking without Regenerative/16(Tq_RR)
  "Tq_RL_wc "/1 -> Braking with Regenerative/3(Tq_RL_wc), Acelerating and braking without Regenerative/17(Tq_RL)
  Tq_max/1 -> Acelerating and braking without Regenerative/1(Tq_max)
  V_eRL/1 -> Acelerating and braking without Regenerative/3(V_eRL)
  Trans_max_dynamic/1 -> Acelerating and braking without Regenerative/4(Trans_max_dynamic)
  "Trans_max_static "/1 -> Acelerating and braking without Regenerative/5(Trans_max_static)
  Merge2/1 -> Tq_RLout/1
  Merge1/1 -> Tq_RRout/1
  Bp/1 -> If/1
  Reg_enable/1 -> If/2
  V_eRR/1 -> Acelerating and braking without Regenerative/2(V_eRR)
  If/1 -> Braking with Regenerative/Action
  If/2 -> Acelerating and braking without Regenerative/Action
  MaxRegTorque/1 -> Braking with Regenerative/1(MaxRegTorque)
  Tq_FRin/1 -> Acelerating and braking without Regenerative/14(Tq_FR)
  Tq_FLin/1 -> Acelerating and braking without Regenerative/15(Tq_FL)
  ReductionCte_Temperature/1 -> Acelerating and braking without Regenerative/13(ReductionCte_Temperature)
  ReductionCte_Power/1 -> Acelerating and braking without Regenerative/12(ReductionCte_Power)
  TemperatureIGBT/1 -> Acelerating and braking without Regenerative/9(TemperatureIGBT)
  Temperature_limit_IGBT/1 -> Acelerating and braking without Regenerative/8(Temperature_limit_IGBT)
  Power/1 -> Acelerating and braking without Regenerative/7(Power)
  Power_limit/1 -> Acelerating and braking without Regenerative/6(Power_limit)
  Acelerating and braking without Regenerative/2(TQ_RL) -> Merge2/1
  Acelerating and braking without Regenerative/1(TQ_RR) -> Merge1/1
  Braking with Regenerative/1(TQ_RR) -> Merge1/2
  Braking with Regenerative/2(TQ_RL) -> Merge2/2
  TemperatureI_limit_Motor/1 -> Acelerating and braking without Regenerative/10(TemperatureI_limit_Motor)
  TemperatureIMotor/1 -> Acelerating and braking without Regenerative/11(TemperatureMotor)
  Acelerating and braking without Regenerative/4(Flag_Power) -> Flag_Power/1
  Acelerating and braking without Regenerative/3(Flag_Temperature) -> Flag_Temperature/1
  Tq_diff/1 -> Acelerating and braking without Regenerative/18(Tq_diff)

== system Torque_Control_ETR07/VDC/If Action Subsystem/VDC 2018 Complete/Driver // CarBehaviours ==
  Tq_FRin : Inport
  Tq_FLin : Inport  Port=2
  Tq_RRin : Inport  Port=3
  "Tq_RLin " : Inport  Port=4
  Bp : Inport  Port=5
  Ap : Inport  Port=6
  Reg_enable : Inport  Port=7
  Ap_Sat_up : Inport  Port=8
  Ap_Sat_down : Inport  Port=9
  Accelerating : Subsystem  TreatAsAtomicUnit=on
  "Accelerator behaviour " : MATLAB Function  TreatAsAtomicUnit=on
  Braking Conditions : If  NumInputs=3  IfExpression=u1>0 & u2<0.1 & u3==1  ElseIfExpressions=u1>0 & u2<0.1 & u3==0, u1<0.1 & u2<0.1
  Constant : Constant  Value=0
  Constant1 : Constant  Value=0
  Inertia Braking : Subsystem  TreatAsAtomicUnit=on
  Mech_Braking : Subsystem  TreatAsAtomicUnit=on
  Merge : Merge  Inputs=4
  Merge1 : Merge  Inputs=4
  Regenerative+Mech Braking : Subsystem  TreatAsAtomicUnit=on
  Terminator : Terminator
  Terminator1 : Terminator
  Tq_FRout : Outport
  "Tq_FLout " : Outport  Port=2
  Tq_RRout : Outport  Port=3
  Tq_RLout : Outport  Port=4
  out_Throttle : Outport  Port=5
  wires:
  Constant1/1 -> "Tq_FLout "/1
  Constant/1 -> Tq_FRout/1
  Tq_FLin/1 -> Terminator1/1
  Tq_FRin/1 -> Terminator/1
  Merge/1 -> Tq_RRout/1
  Merge1/1 -> Tq_RLout/1
  Bp/1 -> Braking Conditions/1
  Regenerative+Mech Braking/1("Tq_RR ") -> Merge/1
  Mech_Braking/1("Tq_RR ") -> Merge/2
  Inertia Braking/1("Tq_RR ") -> Merge/3
  Accelerating/1("Tq_RR ") -> Merge/4
  Regenerative+Mech Braking/2(Tq_RL) -> Merge1/1
  Mech_Braking/2(Tq_RL) -> Merge1/2
  Inertia Braking/2(Tq_RL) -> Merge1/3
  Accelerating/2(Tq_RL) -> Merge1/4
  Braking Conditions/1 -> Regenerative+Mech Braking/Action
  Braking Conditions/2 -> Mech_Braking/Action
  Braking Conditions/3 -> Inertia Braking/Action
  Braking Conditions/4 -> Accelerating/Action
  Tq_RRin/1 -> Accelerating/2(Tq_RR), Regenerative+Mech Braking/1(RegTq_RR)
  "Tq_RLin "/1 -> Accelerating/3("Tq_RL "), Regenerative+Mech Braking/2(RegTq_RL)
  Reg_enable/1 -> Braking Conditions/3
  Accelerating/3(Out_Throttle) -> out_Throttle/1
  "Accelerator behaviour "/1(throttle) -> Accelerating/1(Throttle), Braking Conditions/2
  Ap/1 -> "Accelerator behaviour "/1(Ap)
  Ap_Sat_up/1 -> "Accelerator behaviour "/2(Ap_Sat_up)
  Ap_Sat_down/1 -> "Accelerator behaviour "/3(Ap_Sat_down)

== system Torque_Control_ETR07/VDC/If Action Subsystem/VDC 2018 Complete/Flags ==
  Flag_CarBehavior : Inport
  Flag_WheelSpin_RR : Inport  Port=2
  Flag_WheelSpin_RL : Inport  Port=3
  Flag_Temperature : Inport  Port=4
  Flag_Power : Inport  Port=5
  Mux : Mux  Inputs=5
  Flags : Outport
  wires:
  Mux/1 -> Flags/1
  Flag_CarBehavior/1 -> Mux/1
  Flag_WheelSpin_RR/1 -> Mux/2
  Flag_WheelSpin_RL/1 -> Mux/3
  Flag_Temperature/1 -> Mux/4
  Flag_Power/1 -> Mux/5

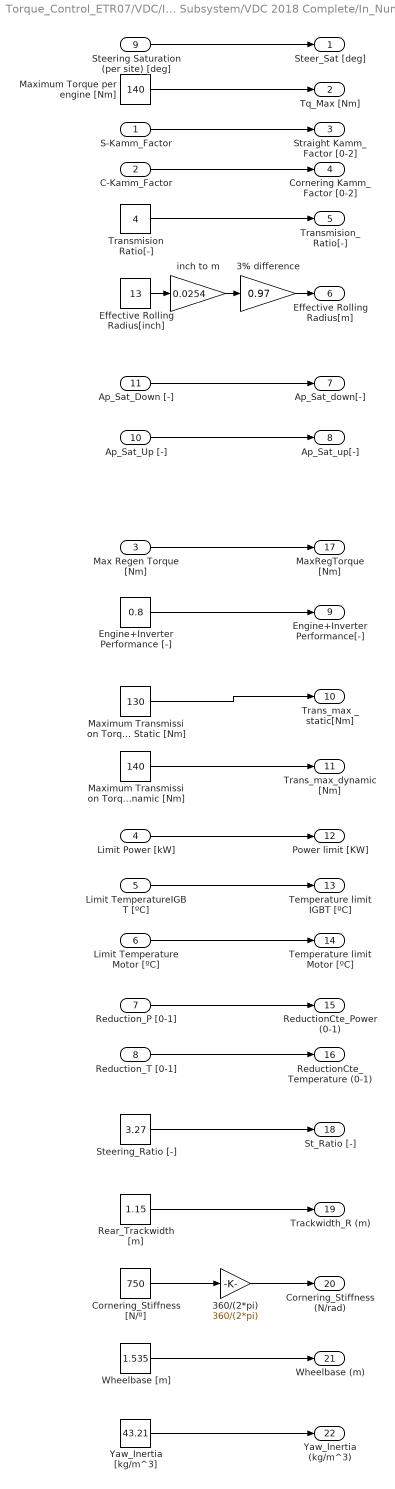
== system Torque_Control_ETR07/VDC/If Action Subsystem/VDC 2018 Complete/In_Numbers ==
  S-Kamm_Factor : Inport
  C-Kamm_Factor : Inport  Port=2
  Max Regen Torque [Nm] : Inport  Port=3
  Limit Power [kW] : Inport  Port=4
  Limit TemperatureIGBT [ºC] : Inport  Port=5
  Limit Temperature Motor [ºC] : Inport  Port=6
  Reduction_P [0-1] : Inport  Port=7
  Reduction_T [0-1] : Inport  Port=8
  Steering Saturation (per site) [deg] : Inport  Port=9
  Ap_Sat_Up [-] : Inport  Port=10
  Ap_Sat_Down [-] : Inport  Port=11
  3% difference : Gain  Gain=0.97
  360/(2*pi) : Gain  Gain=360/(2*pi)
  Cornering_Stiffness [N/º] : Constant  Value=750
  Effective Rolling Radius[inch] : Constant  Value=13
  Engine+Inverter Performance [-] : Constant  Value=0.8
  Maximum Torque per engine [Nm] : Constant  Value=140
  Maximum Transmission Torque Dynamic [Nm] : Constant  Value=140
  Maximum Transmission Torque Static [Nm] : Constant  Value=130
  "Rear_Trackwidth [m] " : Constant  Value=1.15
  Steering_Ratio [-] : Constant  Value=3.27
  Transmision Ratio[-] : Constant  Value=4
  Wheelbase [m] : Constant  Value=1.535
  Yaw_Inertia [kg/m^3] : Constant  Value=43.21  VectorParams1D=off  SampleTime=-1
  inch to m : Gain  Gain=0.0254
  Steer_Sat [deg] : Outport
  Tq_Max [Nm] : Outport  Port=2
  Straight Kamm_Factor [0-2] : Outport  Port=3
  Cornering Kamm_Factor [0-2] : Outport  Port=4
  Transmision_Ratio[-] : Outport  Port=5
  Effective Rolling Radius[m] : Outport  Port=6
  Ap_Sat_down[-] : Outport  Port=7
  Ap_Sat_up[-] : Outport  Port=8
  Engine+Inverter Performance[-] : Outport  Port=9
  Trans_max _static[Nm] : Outport  Port=10
  Trans_max_dynamic [Nm] : Outport  Port=11
  "Power limit [KW] " : Outport  Port=12
  Temperature limit IGBT [ºC] : Outport  Port=13
  Temperature limit Motor [ºC] : Outport  Port=14
  ReductionCte_Power (0-1) : Outport  Port=15
  ReductionCte_Temperature (0-1) : Outport  Port=16
  MaxRegTorque [Nm] : Outport  Port=17
  St_Ratio [-] : Outport  Port=18
  Trackwidth_R (m) : Outport  Port=19
  Cornering_Stiffness (N/rad) : Outport  Port=20
  Wheelbase (m) : Outport  Port=21
  Yaw_Inertia (kg/m^3) : Outport  Port=22
  wires:
  Maximum Torque per engine [Nm]/1 -> Tq_Max [Nm]/1
  Transmision Ratio[-]/1 -> Transmision_Ratio[-]/1
  Effective Rolling Radius[inch]/1 -> inch to m/1
  Maximum Transmission Torque Static [Nm]/1 -> Trans_max _static[Nm]/1
  Maximum Transmission Torque Dynamic [Nm]/1 -> Trans_max_dynamic [Nm]/1
  inch to m/1 -> 3% difference/1
  3% difference/1 -> Effective Rolling Radius[m]/1
  Engine+Inverter Performance [-]/1 -> Engine+Inverter Performance[-]/1
  S-Kamm_Factor/1 -> Straight Kamm_Factor [0-2]/1
  Max Regen Torque [Nm]/1 -> MaxRegTorque [Nm]/1
  Limit Power [kW]/1 -> "Power limit [KW] "/1
  Limit TemperatureIGBT [ºC]/1 -> Temperature limit IGBT [ºC]/1
  Reduction_P [0-1]/1 -> ReductionCte_Power (0-1)/1
  C-Kamm_Factor/1 -> Cornering Kamm_Factor [0-2]/1
  Steering Saturation (per site) [deg]/1 -> Steer_Sat [deg]/1
  Ap_Sat_Up [-]/1 -> Ap_Sat_up[-]/1
  Ap_Sat_Down [-]/1 -> Ap_Sat_down[-]/1
  Reduction_T [0-1]/1 -> ReductionCte_Temperature (0-1)/1
  Limit Temperature Motor [ºC]/1 -> Temperature limit Motor [ºC]/1
  Steering_Ratio [-]/1 -> St_Ratio [-]/1
  "Rear_Trackwidth [m] "/1 -> Trackwidth_R (m)/1
  Cornering_Stiffness [N/º]/1 -> 360/(2*pi)/1
  Wheelbase [m]/1 -> Wheelbase (m)/1
  360/(2*pi)/1 -> Cornering_Stiffness (N/rad)/1
  Yaw_Inertia [kg/m^3]/1 -> Yaw_Inertia (kg/m^3)/1

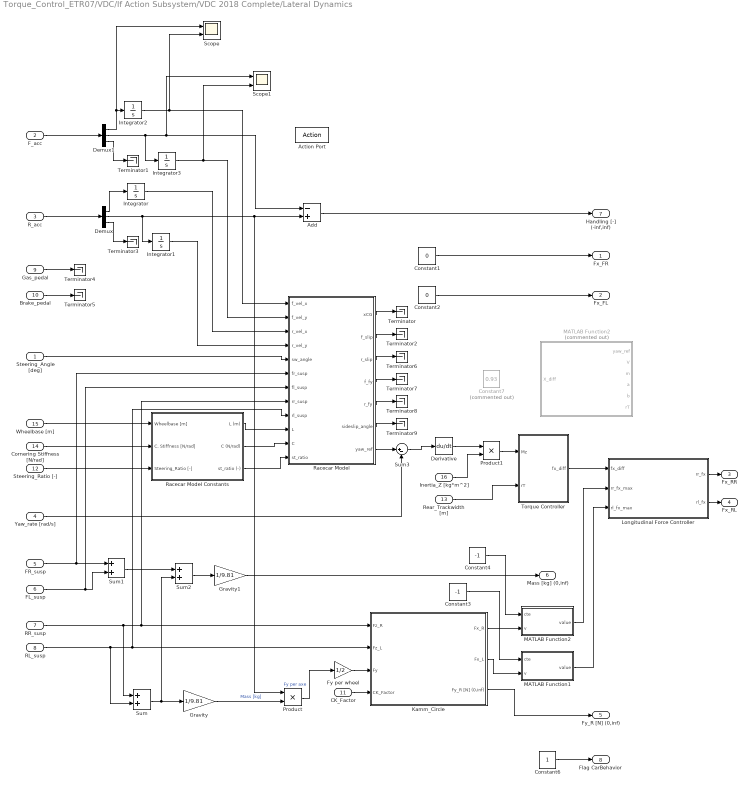
== system Torque_Control_ETR07/VDC/If Action Subsystem/VDC 2018 Complete/Lateral Dynamics ==
  Steering_Angle [deg] : Inport
  F_acc : Inport  Port=2
  R_acc : Inport  Port=3
  Yaw_rate [rad/s] : Inport  Port=4
  FR_susp : Inport  Port=5
  FL_susp : Inport  Port=6
  RR_susp : Inport  Port=7
  RL_susp : Inport  Port=8
  Gas_pedal : Inport  Port=9
  Brake_pedal : Inport  Port=10
  CK_Factor : Inport  Port=11
  Steering_Ratio [-] : Inport  Port=12
  Rear_Trackwidth [m] : Inport  Port=13
  Cornering Stiffness [N/rad] : Inport  Port=14
  Wheelbase [m] : Inport  Port=15
  Inertia_Z [kg*m^2] : Inport  Port=16
  Action Port : ActionPort  ActionType=else
  Add : Sum  Inputs=-+
  Constant1 : Constant  Value=0
  Constant2 : Constant  Value=0
  Constant3 : Constant  Value=-1
  Constant4 : Constant  Value=-1
  Constant6 : Constant
  Constant7 : Constant  Commented=on  Value=0.93
  Demux : Demux  Outputs=3
  Demux1 : Demux  Outputs=3
  Derivative : Derivative
  Fy per wheel : Gain  Gain=1/2
  Gravity : Gain  Gain=1/9.81
  Gravity1 : Gain  Gain=1/9.81
  Integrator{,1..3} (4 alike) : Integrator
  Kamm_Circle : Subsystem
  Longitudinal Force Controller : MATLAB Function  TreatAsAtomicUnit=on
  MATLAB Function1 : MATLAB Function  TreatAsAtomicUnit=on
  MATLAB Function2 : MATLAB Function  TreatAsAtomicUnit=on
  "MATLAB Function2 " : MATLAB Function  Commented=on  TreatAsAtomicUnit=on
  Product : Product
  Product1 : Product
  Racecar Model : MATLAB Function  TreatAsAtomicUnit=on
  Racecar Model Constants : Subsystem
  Scope : Scope  NumInputPorts=2
  Scope1 : Scope  NumInputPorts=2
  Sum : Sum
  Sum1 : Sum
  Sum2 : Sum
  Sum3 : Sum  Inputs=|+-
  Terminator{,1..9} (10 alike) : Terminator
  Torque Controller : MATLAB Function  TreatAsAtomicUnit=on
  Fx_FR : Outport
  Fx_FL : Outport  Port=2
  "Fx_RR " : Outport  Port=3
  "Fx_RL " : Outport  Port=4
  Fy_R [N] (0,inf) : Outport  Port=5
  " Mass [kg] (0,inf)" : Outport  Port=6
  Handling [-] (-inf,inf) : Outport  Port=7
  Flag CarBehavior : Outport  Port=8
  wires:
  Gas_pedal/1 -> Terminator4/1
  Brake_pedal/1 -> Terminator5/1
  R_acc/1 -> Demux/1
  Demux/2 -> Integrator1/1, Add/2, Product/1
  Demux/1 -> Integrator/1
  Demux/3 -> Terminator3/1
  Product/1 -> Fy per wheel/1  "Fy per axe"
  Constant1/1 -> Fx_FR/1
  Constant2/1 -> Fx_FL/1
  RR_susp/1 -> Racecar Model/8(rr_susp), Kamm_Circle/1(Fz_R), Sum/1
  RL_susp/1 -> Racecar Model/9(rl_susp), Kamm_Circle/2(Fz_L), Sum/2
  Fy per wheel/1 -> Kamm_Circle/3(Fy)
  CK_Factor/1 -> Kamm_Circle/4(CK_Factor)
  Kamm_Circle/3(Fy_R [N] (0,inf)) -> Fy_R [N] (0,inf)/1
  Sum/1 -> Gravity/1, Sum2/2
  Gravity/1 -> Product/2  "Mass [kg]"
  FR_susp/1 -> Racecar Model/6(fr_susp), Sum1/1
  FL_susp/1 -> Racecar Model/7(fl_susp), Sum1/2
  Sum1/1 -> Sum2/1
  Sum2/1 -> Gravity1/1
  Gravity1/1 -> " Mass [kg] (0,inf)"/1
  F_acc/1 -> Demux1/1
  Demux1/3 -> Terminator1/1
  Add/1 -> Handling [-] (-inf,inf)/1
  Demux1/2 -> Integrator3/1, Scope1/1, Add/1
  Constant3/1 -> MATLAB Function1/1(cte)
  Constant4/1 -> MATLAB Function2/1(cte)
  Kamm_Circle/1(Fx_R) -> MATLAB Function2/2(v)
  Kamm_Circle/2(Fx_L) -> MATLAB Function1/2(v)
  Constant6/1 -> Flag CarBehavior/1
  MATLAB Function2/1(value) -> Longitudinal Force Controller/2(rr_fx_max)
  MATLAB Function1/1(value) -> Longitudinal Force Controller/3(rl_fx_max)
  Longitudinal Force Controller/2(rl_fx) -> "Fx_RL "/1
  Longitudinal Force Controller/1(rr_fx) -> "Fx_RR "/1
  Wheelbase [m]/1 -> Racecar Model Constants/1(Wheelbase [m])
  Cornering Stiffness [N/rad]/1 -> Racecar Model Constants/2(C. Stiffness [N/rad])
  Steering_Ratio [-]/1 -> Racecar Model Constants/3(Steering_Ratio [-])
  Steering_Angle [deg]/1 -> Racecar Model/5(sw_angle)
  Integrator2/1 -> Scope/2, Racecar Model/1(f_vel_x)
  Integrator3/1 -> Scope1/2, Racecar Model/2(f_vel_y)
  Integrator/1 -> Racecar Model/3(r_vel_x)
  Integrator1/1 -> Racecar Model/4(r_vel_y)
  Racecar Model Constants/3(st_ratio (-)) -> Racecar Model/12(st_ratio)
  Racecar Model Constants/2(C (N/rad)) -> Racecar Model/11(C)
  Racecar Model Constants/1(L (m)) -> Racecar Model/10(L)
  Racecar Model/6(sideslip_angle) -> Terminator9/1
  Racecar Model/5(r_fy) -> Terminator8/1
  Racecar Model/4(f_fy) -> Terminator7/1
  Racecar Model/3(r_slip) -> Terminator6/1
  Racecar Model/2(f_slip) -> Terminator2/1
  Racecar Model/1(xCG) -> Terminator/1
  Yaw_rate [rad/s]/1 -> Sum3/2
  Racecar Model/7(yaw_ref) -> Sum3/1
  Sum3/1 -> Derivative/1
  Derivative/1 -> Product1/1
  Inertia_Z [kg*m^2]/1 -> Product1/2
  Rear_Trackwidth [m]/1 -> Torque Controller/2(rT)
  Product1/1 -> Torque Controller/1(Mz)
  Torque Controller/1(fx_diff) -> Longitudinal Force Controller/1(fx_diff)
  Demux1/1 -> Integrator2/1, Scope/1
